simulink model "fmcw_dechirp_test"  (R2025b)
settings: Solver=FixedStepDiscrete  StartTime=0.0  StopTime=5.115e-06  FixedStep=5e-09  RelTol=1e-3
settings Model: DataTypeOverride=Off  Creator=kimsteph  LastModifiedBy=kimsteph
settings OptimizationCC: BlockReduction=off  ConditionallyExecuteInputs=off  DefaultParameterBehavior=Inlined  InheritOutputTypeSmallerThanSingle=on
settings DebuggingCC: ArtificialAlgebraicLoopMsg=error  SingleTaskRateTransMsg=error
settings HardwareCC: ProdBitPerPointer=32.0  ProdBitPerSizeT=32.0  ProdBitPerPtrDiffT=32.0  ProdLargestAtomicFloat=None  ProdIntDivRoundTo=Undefined  ProdEndianess=Unspecified  ProdWordSize=32.0  ProdHWDeviceType=ASIC/FPGA->ASIC/FPGA  TargetBitPerPointer=64.0  TargetBitPerSizeT=64.0  TargetBitPerPtrDiffT=64.0  TargetLongLongMode=on  TargetIntDivRoundTo=Zero  TargetEndianess=LittleEndian  TargetWordSize=64.0  TargetHWDeviceType=Custom Processor->MATLAB Host Computer  ProdEqTarget=off

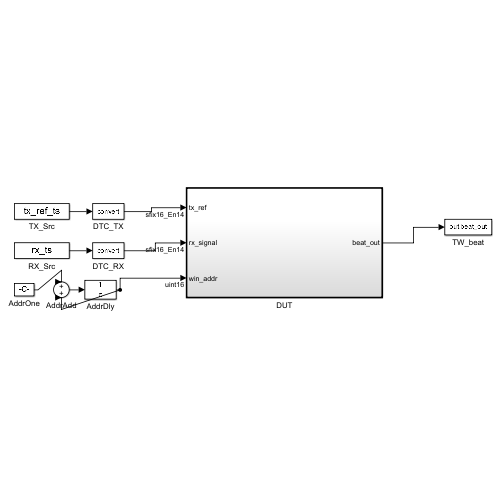
[thumbnail: Simulink's stored preview of the top-level diagram]
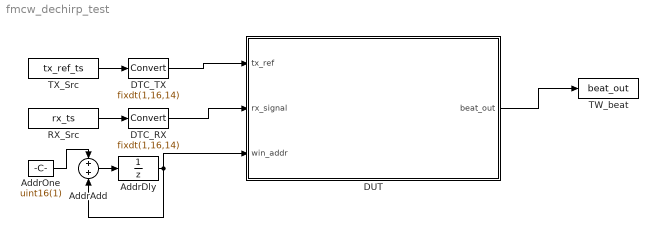
== system fmcw_dechirp_test ==
  AddrAdd : Sum  OutDataTypeStr=uint16
  AddrDly : UnitDelay  SampleTime=5e-09  HasFrameUpgradeWarning=on
  AddrOne : Constant  Value=uint16(1)  OutDataTypeStr=uint16
  DTC_RX : DataTypeConversion  OutDataTypeStr=fixdt(1,16,14)  RndMeth=Nearest  SaturateOnIntegerOverflow=off
  DTC_TX : DataTypeConversion  OutDataTypeStr=fixdt(1,16,14)  RndMeth=Nearest  SaturateOnIntegerOverflow=off
  DUT : Subsystem  TreatAsAtomicUnit=on
  RX_Src : FromWorkspace  VariableName=rx_ts
  TW_beat : ToWorkspace  VariableName=beat_out  SaveFormat=Timeseries  SampleTime=-1
  TX_Src : FromWorkspace  VariableName=tx_ref_ts
  wires:
  AddrOne/1 -> AddrAdd/1
  AddrDly/1 -> AddrAdd/2, DUT/3(win_addr)
  AddrAdd/1 -> AddrDly/1
  TX_Src/1 -> DTC_TX/1
  RX_Src/1 -> DTC_RX/1
  DTC_TX/1 -> DUT/1(tx_ref)
  DTC_RX/1 -> DUT/2(rx_signal)
  DUT/1(beat_out) -> TW_beat/1

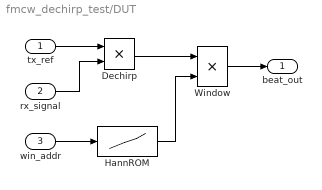
== system fmcw_dechirp_test/DUT ==
  tx_ref : Inport  OutDataTypeStr=fixdt(1,16,14)
  rx_signal : Inport  Port=2  OutDataTypeStr=fixdt(1,16,14)
  win_addr : Inport  Port=3  OutDataTypeStr=uint16
  Dechirp : Product  OutDataTypeStr=fixdt(1,16,14)
  HannROM : Lookup_n-D  NumberOfTableDimensions=1  BreakpointsForDimension1=[0 1 2 3 4 5 6 7 8 9 10 11 12 13 14 15 16 17 18 19 20 21 22 23 24 25 26 27 28 29 30 31 32 33 34 35 36 37 38 39 40 41 42 43 44 45 46 47 48 49 50 51 52 53 54 55 56 57 58 59 60 61 62 63 64 65 66 67 68 69 70 71 72 73 74 75 76 77 78 79 80 81 82 83 84 85 86 87 88 89 90 91 92 93 94 95 96 97 98 99 100 101 102 103 104 105 106 107 108 109 110 111 112 113 114 115 116 117 118 119 120 121 122 123 124 125 126 127 128 129 130 131 132 133 134 135 136 137 138 139 140 141 142 143 144 145 146 147 148 149 150 151 152 153 154 155 156 157 158 159 160 161 162 163 164 165 166 167 168 169 170 171 172 173 174 175 176 177 178 179 180 181 182 183 184 185 186 187 188 189 190 191 192 193 194 195 196 197 198 199 200 201 202 203 204 205 206 207 208 209 210 211 212 213 214 215 216 217 218 219 220 221 222 223 224 225 226 227 228 229 230 231 232 233 234 235 236 237 238 239 240 241 242 243 244 245 246 247 248 249 250 251 252 253 254 255 256 257 258 259 260 261 262 263 264 265 266 267 268 269 270 271 272 273 274 275 276 277 278 279 280 281 282 283 284 285 286 287 288 289 290 291 292 293 294 295 296 297 298 299 300 301 302 303 304 305 306 307 308 309 310 311 312 313 314 315 316 317 318 319 320 321 322 323 324 325 326 327 328 329 330 331 332 333 334 335 336 337 338 339 340 341 342 343 344 345 346 347 348 349 350 351 352 353 354 355 356 357 358 359 360 361 362 363 364 365 366 367 368 369 370 371 372 373 374 375 376 377 378 379 380 381 382 383 384 385 386 387 388 389 390 391 392 393 394 395 396 397 398 399 400 401 402 403 404 405 406 407 408 409 410 411 412 413 414 415 416 417 418 419 420 421 422 423 424 425 426 427 428 429 430 431 432 433 434 435 436 437 438 439 440 441 442 443 444 445 446 447 448 449 450 451 452 453 454 455 456 457 458 459 460 461 462 463 464 465 466 467 468 469 470 471 472 473 474 475 476 477 478 479 480 481 482 483 484 485 486 487 488 489 490 491 492 493 494 495 496 497 498 499 500 501 502 503 504 505 506 507 508 509 510 511 512 513 514 515 516 517 518 519 520 521 522 523 524 525 526 527 528 529 530 531 532 533 534 535 536 537 538 539 540 541 542 543 544 545 546 547 548 549 550 551 552 553 554 555 556 557 558 559 560 561 562 563 564 565 566 567 568 569 570 571 572 573 574 575 576 577 578 579 580 581 582 583 584 585 586 587 588 589 590 591 592 593 594 595 596 597 598 599 600 601 602 603 604 605 606 607 608 609 610 611 612 613 614 615 616 617 618 619 620 621 622 623 624 625 626 627 628 629 630 631 632 633 634 635 636 637 638 639 640 641 642 643 644 645 646 647 648 649 650 651 652 653 654 655 656 657 658 659 660 661 662 663 664 665 666 667 668 669 670 671 672 673 674 675 676 677 678 679 680 681 682 683 684 685 686 687 688 689 690 691 692 693 694 695 696 697 698 699 700 701 702 703 704 705 706 707 708 709 710 711 712 713 714 715 716 717 718 719 720 721 722 723 724 725 726 727 728 729 730 731 732 733 734 735 736 737 738 739 740 741 742 743 744 745 746 747 748 749 750 751 752 753 754 755 756 757 758 759 760 761 762 763 764 765 766 767 768 769 770 771 772 773 774 775 776 777 778 779 780 781 782 783 784 785 786 787 788 789 790 791 792 793 794 795 796 797 798 799 800 801 802 803 804 805 806 807 808 809 810 811 812 813 814 815 816 817 818 819 820 821 822 823 824 825 826 827 828 829 830 831 832 833 834 835 836 837 838 839 840 841 842 843 844 845 846 847 848 849 850 851 852 853 854 855 856 857 858 859 860 861 862 863 864 865 866 867 868 869 870 871 872 873 874 875 876 877 878 879 880 881 882 883 884 885 886 887 888 889 890 891 892 893 894 895 896 897 898 899 900 901 902 903 904 905 906 907 908 909 910 911 912 913 914 915 916 917 918 919 920 921 922 923 924 925 926 927 928 929 930 931 932 933 934 935 936 937 938 939 940 941 942 943 944 945 946 947 948 949 950 951 952 953 954 955 956 957 958 959 960 961 962 963 964 965 966 967 968 969 970 971 972 973 974 975 976 977 978 979 980 981 982 983 984 985 986 987 988 989 990 991 992 993 994 995 996 997 998 999 1000 1001 1002 1003 1004 1005 1006 1007 1008 1009 1010 1011 1012 1013 1014 1015 1016 1017 1018 1019 1020 1021 1022 1023]  Table=[0;9.43077e-06;3.77227e-05;8.48748e-05;0.000150885;0.000235751;0.00033947;0.000462038;0.00060345;0.0007637;0.000942783;0.00114069;0.00135742;0.00159296;0.0018473;0.00212043;0.00241234;0.00272303;0.00305247;0.00340066;0.00376758;0.00415322;0.00455757;0.0049806;0.00542231;0.00588268;0.00636168;0.00685931;0.00737554;0.00791036;0.00846373;0.00903565;0.00962609;0.010235;0.0108624;0.0115083;0.0121726;0.0128553;0.0135564;0.0142758;0.0150135;0.0157696;0.0165439;0.0173364;0.0181472;0.0189761;0.0198232;0.0206884;0.0215716;0.022473;0.0233923;0.0243296;0.0252849;0.026258;0.027249;0.0282579;0.0292846;0.030329;0.0313911;0.0324709;0.0335684;0.0346834;0.035816;0.0369661;0.0381337;0.0393187;0.0405211;0.0417408;0.0429778;0.044232;0.0455035;0.046792;0.0480977;0.0494204;0.0507602;0.0521168;0.0534904;0.0548808;0.056288;0.0577119;0.0591525;0.0606098;0.0620836;0.0635739;0.0650807;0.0666039;0.0681435;0.0696993;0.0712714;0.0728597;0.0744641;0.0760845;0.0777209;0.0793732;0.0810414;0.0827255;0.0844252;0.0861406;0.0878717;0.0896183;0.0913804;0.0931578;0.0949507;0.0967588;0.0985821;0.100421;0.102274;0.104143;0.106026;0.107924;0.109838;0.111765;0.113708;0.115665;0.117637;0.119623;0.121623;0.123638;0.125666;0.127709;0.129766;0.131837;0.133922;0.136021;0.138133;0.140259;0.142399;0.144552;0.146718;0.148898;0.151091;0.153297;0.155517;0.157749;0.159994;0.162252;0.164523;0.166806;0.169102;0.171411;0.173732;0.176065;0.17841;0.180768;0.183137;0.185519;0.187912;0.190317;0.192734;0.195163;0.197603;0.200054;0.202517;0.20499;0.207476;0.209972;0.212479;0.214996;0.217525;0.220064;0.222614;0.225174;0.227745;0.230326;0.232917;0.235518;0.238129;0.24075;0.243381;0.246021;0.248671;0.251331;0.254;0.256678;0.259365;0.262062;0.264767;0.267482;0.270205;0.272936;0.275677;0.278425;0.281183;0.283948;0.286721;0.289503;0.292292;0.29509;0.297895;0.300708;0.303528;0.306355;0.30919;0.312033;0.314882;0.317738;0.320601;0.323471;0.326347;0.32923;0.33212;0.335016;0.337918;0.340826;0.34374;0.34666;0.349586;0.352518;0.355455;0.358397;0.361345;0.364298;0.367256;0.37022;0.373188;0.376161;0.379138;0.382121;0.385107;0.388098;0.391093;0.394092;0.397096;0.400103;0.403114;0.406128;0.409146;0.412168;0.415193;0.418221;0.421252;0.424286;0.427323;0.430363;0.433405;0.43645;0.439497;0.442547;0.445598;0.448652;0.451708;0.454765;0.457824;0.460885;0.463948;0.467011;0.470076;0.473142;0.476209;0.479277;0.482346;0.485415;0.488485;0.491555;0.494626;0.497697;0.500768;0.503839;0.506909;0.50998;0.51305;0.51612;0.519189;0.522257;0.525325;0.528391;0.531457;0.534521;0.537584;0.540645;0.543705;0.546764;0.54982;0.552875;0.555928;0.558978;0.562027;0.565073;0.568116;0.571157;0.574196;0.577231;0.580264;0.583294;0.58632;0.589343;0.592363;0.595379;0.598392;0.601401;0.604406;0.607408;0.610405;0.613398;0.616387;0.619371;0.622351;0.625326;0.628297;0.631263;0.634223;0.637179;0.640129;0.643075;0.646015;0.648949;0.651878;0.654801;0.657718;0.660629;0.663534;0.666433;0.669326;0.672212;0.675092;0.677965;0.680831;0.683691;0.686544;0.689389;0.692228;0.695059;0.697883;0.7007;0.703509;0.70631;0.709103;0.711889;0.714666;0.717436;0.720197;0.72295;0.725695;0.728431;0.731158;0.733877;0.736587;0.739288;0.741979;0.744662;0.747336;0.75;0.752655;0.7553;0.757936;0.760562;0.763178;0.765784;0.76838;0.770966;0.773542;0.776107;0.778662;0.781207;0.783741;0.786264;0.788776;0.791278;0.793768;0.796248;0.798716;0.801173;0.803619;0.806053;0.808476;0.810887;0.813286;0.815673;0.818049;0.820413;0.822764;0.825103;0.82743;0.829745;0.832047;0.834337;0.836614;0.838879;0.84113;0.843369;0.845595;0.847808;0.850007;0.852194;0.854367;0.856527;0.858673;0.860806;0.862925;0.86503;0.867122;0.8692;0.871264;0.873314;0.87535;0.877372;0.879379;0.881372;0.883351;0.885315;0.887265;0.8892;0.891121;0.893027;0.894917;0.896793;0.898655;0.900501;0.902331;0.904147;0.905948;0.907733;0.909503;0.911257;0.912996;0.914719;0.916427;0.918119;0.919795;0.921455;0.923099;0.924728;0.92634;0.927936;0.929517;0.931081;0.932628;0.93416;0.935675;0.937173;0.938655;0.940121;0.94157;0.943002;0.944418 ...(+5372 chars)]  InterpMethod=Flat  InternalRulePriority=Speed  OutDataTypeStr=fixdt(0,16,16)  RndMeth=Simplest
  Window : Product  OutDataTypeStr=fixdt(1,16,14)
  beat_out : Outport
  wires:
  tx_ref/1 -> Dechirp/1
  HannROM/1 -> Window/2
  rx_signal/1 -> Dechirp/2
  win_addr/1 -> HannROM/1
  Dechirp/1 -> Window/1
  Window/1 -> beat_out/1
